simulink model "taketwo_single_sim"  (R2025a)
settings: Solver=VariableStepAuto  StartTime=0.0  StopTime=60  RelTol=1e-3
model workspace (MAT data in the model file):
  modeVal = [0; 1; 2; 3]
settings Model: Creator=katiegildersleeve  LastModifiedBy=jennamalone
settings DebuggingCC: UnderSpecifiedDimensionMsg=warning

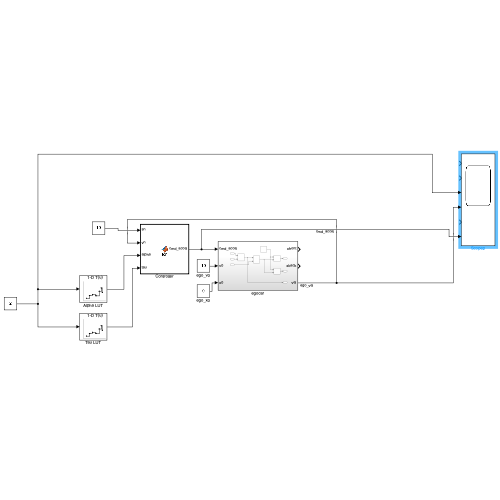
[thumbnail: Simulink's stored preview of the top-level diagram]
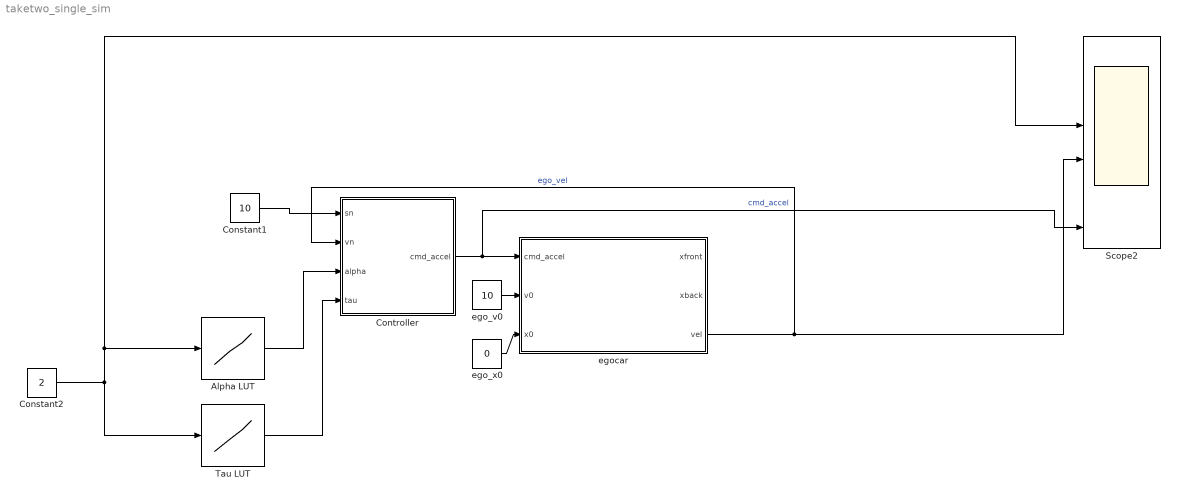
== system taketwo_single_sim ==
  Alpha LUT : Lookup_n-D  NumberOfTableDimensions=1  BreakpointsForDimension1=[0 1 2 3]  Table=[0.75 0.75 1.0 0.25]  InterpMethod=Nearest  InternalRulePriority=Speed  RndMeth=Simplest
  Constant1 : Constant  Value=10
  Constant2 : Constant  Value=2
  Controller : MATLAB Function  TreatAsAtomicUnit=on
  Scope2 : Scope  NumInputPorts=6
      settings: ActiveDisplayYMinimum=-24.985365760598057  ActiveDisplayYMaximum=65.782760720813286
  Tau LUT : Lookup_n-D  NumberOfTableDimensions=1  BreakpointsForDimension1=[0 1 2 3]  Table=[0.75 0.75 0.5 3.0]  InterpMethod=Nearest  InternalRulePriority=Speed  RndMeth=Simplest
  ego_v0 : Constant  Value=10
  ego_x0 : Constant  Value=0
  egocar : Subsystem
  wires:
  ego_v0/1 -> egocar/2(v0)
  egocar/3(vel) -> Controller/2(vn), Scope2/4  "ego_vel"
  ego_x0/1 -> egocar/3(x0)
  Tau LUT/1 -> Controller/4(tau)
  Alpha LUT/1 -> Controller/3(alpha)
  Constant2/1 -> Tau LUT/1, Scope2/3, Alpha LUT/1
  Controller/1(cmd_accel) -> Scope2/6, egocar/1(cmd_accel)  "cmd_accel"
  Constant1/1 -> Controller/1(sn)

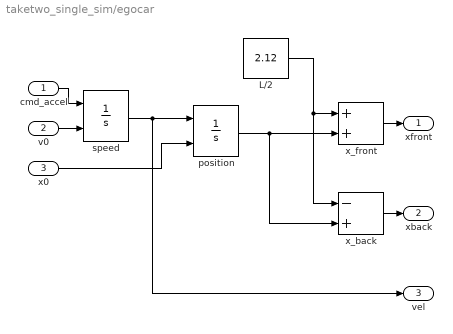
== system taketwo_single_sim/egocar ==
  cmd_accel : Inport
  v0 : Inport  Port=2
  x0 : Inport  Port=3
  L/2 : Constant  Value=2.12
  position : Integrator  InitialConditionSource=external
  speed : Integrator  InitialConditionSource=external
  x_back : Sum  Inputs=-+
  x_front : Sum
  xfront : Outport
  xback : Outport  Port=2
  vel : Outport  Port=3
  wires:
  v0/1 -> speed/2
  x0/1 -> position/2
  cmd_accel/1 -> speed/1
  x_front/1 -> xfront/1
  x_back/1 -> xback/1
  position/1 -> x_back/2, x_front/2
  speed/1 -> vel/1, position/1
  L/2/1 -> x_back/1, x_front/1

== matlab function taketwo_single_sim/Controller ==
  data: sn input; vn input; cmd_accel output; alpha input; tau input
function cmd_accel = fcn(sn, vn, alpha, tau)
% sn   : space gap [m]
% vn   : ego velocity [m/s]
% dv   : relative velocity (v_lead - v_ego) [m/s]
% alpha: gain on space gap error [1/s^2]
% beta : gain on relative velocity [1/s]
% tau  : time gap [s]

    % PD-like control: combine space-gap error and relative velocity
    a = alpha * (sn - tau * vn);

    % clamp acceleration to safe range [-3, 1.5]
    if a < -3.0
        cmd_accel = -3.0;
    elseif a > 1.5
        cmd_accel = 1.5;
    else
        cmd_accel = a;
    end
end
